simulink model "CustomLidarSLAM"  (R2024a)
settings: Solver=VariableStepAuto  StartTime=0.0  StopTime=30  RelTol=1e-3
model workspace (MAT data in the model file):
  IMUloc = [0 0 0]
values from neighbouring files (symbols this model uses):
  refPosesT = [timeVector, smoothRefPoses(:,3)]    [lidar_slam_project.m]    (also in lidar_slam_script.m)
  refPosesX = [timeVector, smoothRefPoses(:,1)]    [lidar_slam_project.m]    (also in lidar_slam_script.m)
  refPosesY = [timeVector, smoothRefPoses(:,2)]    [lidar_slam_project.m]    (also in lidar_slam_script.m)
undefined symbols (not defined in the file or in its folder): Sim3dSensor
libraries: vehdynlibsens x1, sim3dphyssensorlib x1, sim3dlib x1, sim3dautolib x1
settings Model: Creator=The MathWorks, Inc.  LastModifiedBy=FilippoOttaviani
settings SolverCC: AlgebraicLoopSolver=TrustRegion
settings DebuggingCC: UnconnectedInputMsg=warning  UnconnectedOutputMsg=warning  UnconnectedLineMsg=warning  SymbolicDimsDataTypeCodeGenerationDiagnostic=none
settings ModelReferenceCC: EnableRefExpFcnMdlSchedulingChecks=on
settings RTWCC: GPUComputeCapability=3.5  DLArmComputeVersion=19.05

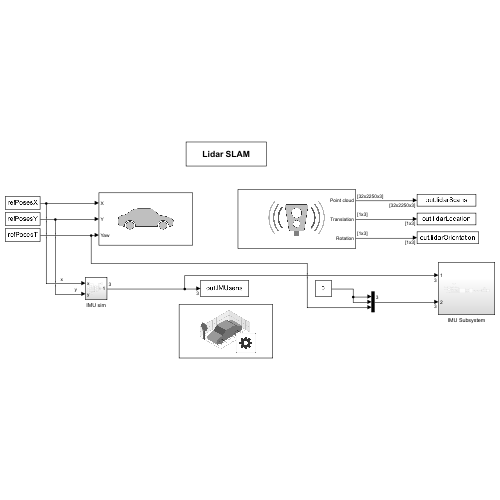
[thumbnail: Simulink's stored preview of the top-level diagram]
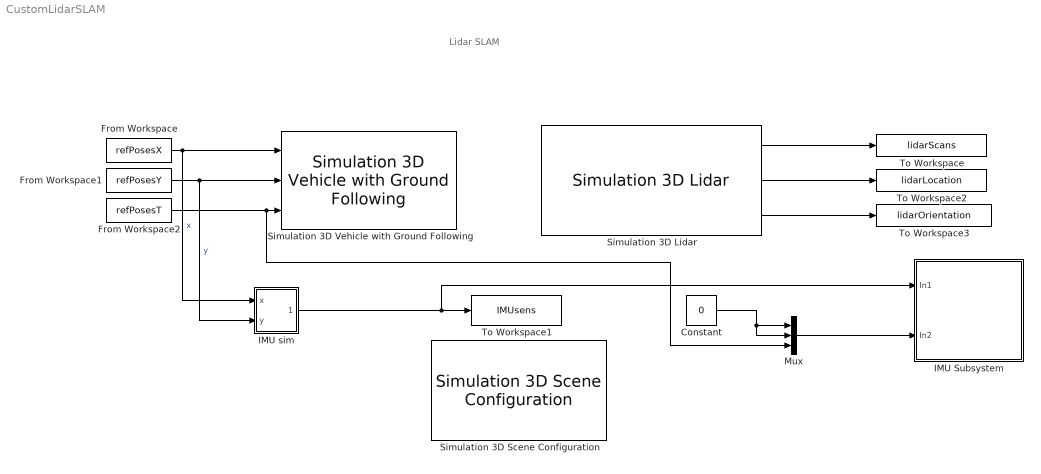
== system CustomLidarSLAM ==
  note: Lidar SLAM
  Constant : Constant  Value=0
  From Workspace : FromWorkspace  VariableName=refPosesX
  From Workspace1 : FromWorkspace  VariableName=refPosesY
  From Workspace2 : FromWorkspace  VariableName=refPosesT  Interpolate=off  OutputAfterFinalValue=Holding final value
  IMU Subsystem : Subsystem
  IMU sim : Subsystem
  Mux : Mux  Inputs=3
  Simulation 3D Lidar : sim3dphyssensorlib/Simulation 3D Lidar  Priority=1  sensorTag=Sim3dSensor�  sensorId=1  sensorName=Sim3dSensor�  vehTagList={'Scene Origin';'SimulinkVehicle1'}  vehTag=SimulinkVehicle1  mountLoc=Roof center  offsetFlag=off  tmountOffset=[0, 0, 0]  rmountOffset=[0, 0, 0]  DetectionRange=100  RangeResolution=0.02  VerticalFOV=40  VerticalResolution=1.25  HorizontalFOV=360  HorizontalResolution=0.16  DistanceOutportEnabled=off  ReflectivityOutportEnabled=off  SemanticOutportEnabled=off  TransformOutportEnabled=on  SampleTime=-1  mountPoint=[-0.25 0 1.57000005245209]  mountOrientation=[0 0 0]  aMode=5  ID=1
      settings: LibrarySourceBlock=sl3dlib/Simulation 3D/Sensors/Simulation 3D Lidar
  Simulation 3D Scene Configuration : sim3dlib/Simulation 3D Scene Configuration  Priority=0  ProjectFormat=Default Scenes  SceneDesc=US city block  ProjectName=C:\Program Files\MATLAB\R2024a\toolbox\shared\sim3d_projects\automotive_project_windows\UE\WindowsNoEditor\VehicleSimulation.exe  ScenePath=/Game/Maps/HwStrght  EnableOpenDRIVE=off  vehTagList={'Custom';'Scene Origin';'SimulinkVehicle1'}  vehTag=SimulinkVehicle1  FreeCameraInitialTranslation=[0, 0, 0]  FreeCameraDefaultInitialTranslation=[-6, 0, 2]  FreeCameraInitialRotation=[0, 0, 0]  FreeCameraDefaultInitialRotation=[0, -15, 0]  OpVisEn=off  Ts=1/60  EnableWindow=on  EnableRemoteAccess=off  EnableWeather=off  SunAzimuth=90  SunAltitude=40.0  EnableGeospatialSun=off  Latitude=0  Longitude=0  Date=2023-01-01  Time=10:30:00  GeoTimeZone=-5.0  SunDaylightSaving=off  wind=1  clouds=10  EnableVolumetricClouds=off  CloudCoverage=0  CloudAltitude=6  fog=0  rain=0  RaindropsEffect=off  SnowDensity=0  EnableGeospatial=off  UseTrueOrigin=off  OriginHeight=200  OriginLatitude=40.744652  OriginLongitude=-73.988864  MapStyle=Aerial  AdditionalAssetIDs=[]  UseAdvancedSunSky=off  SolarTime=11  TimeZone=-5  Day=21  Month=9  Year=2022  UseDaylightSavingTime=on  DSTStartDay=10  DSTStartMonth=3  DSTEndDay=3  DSTEndMonth=11  DSTSwitchHour=2  sensorTag=MainCamera2  sensorId=2  sensorName=MainCamera2  mountLoc=Origin  offsetFlag=off  tmountOffset=[0, 0, 0]  rmountOffset=[0, 0, 0]  HorizontalResolution=1280  VerticalResolution=720  HorizontalFOV=60  mountPoint=[0 0 0]  mountOrientation=[0 0 0]  aMode=3  ID=2  GeoTrigger=Inactive
      settings: LibrarySourceBlock=drivingsim3d/Simulation 3D Scene Configuration
  Simulation 3D Vehicle with Ground Following : sim3dautolib/Simulation 3D Vehicle with Ground Following  Priority=-1  PassVehMesh=Muscle car  MeshPath=/MathWorksSimulation/Vehicles/Muscle/Meshes/SK_MuscleCar.SK_MuscleCar  TrackWidth=1.9  WheelBase=3  WheelRadius=0.35  VehColor=Black  InitialPos=[refPosesX(1,2), refPosesY(1,2), 0]  InitialRot=[0, 0, refPosesT(1,2)]  ActorName=SimulinkVehicle1  SampleTime=-1  ActorType=SimulinkVehicle  ID=1  aMode=3  ActorTag=SimulinkVehicle1  CoordinateScheme=ISO  VehLightsControl=off  HeadlightColor=[ 1, 1, 1 ]  HighBeamIntensity=100000  LowBeamIntensity=60000  HighBeamConeAngle=70  LowBeamConeAngle=70  LeftHeadlightOrientation=[ 0, 0 ]  RightHeadlightOrientation=[ 0, 0 ]  BrakelightIntensity=500  ReverselightIntensity=500  SignallightIntensity=500  SignallightPeriod=1  SignalPulseWidth=50  TransformOutportEnabled=off
      settings: LibrarySourceBlock=drivingsim3d/Simulation 3D Vehicle with Ground Following
  To Workspace : ToWorkspace  VariableName=lidarScans  SaveFormat=Structure With Time  SampleTime=0.1
  To Workspace1 : ToWorkspace  VariableName=IMUsens  SaveFormat=Timeseries  SampleTime=-1
  To Workspace2 : ToWorkspace  VariableName=lidarLocation  SaveFormat=Structure With Time  SampleTime=0.1
  To Workspace3 : ToWorkspace  VariableName=lidarOrientation  SaveFormat=Structure With Time  SampleTime=0.1
  wires:
  From Workspace/1 -> IMU sim/1(x), Simulation 3D Vehicle with Ground Following/1  "x"
  From Workspace1/1 -> IMU sim/2(y), Simulation 3D Vehicle with Ground Following/2  "y"
  From Workspace2/1 -> Mux/3, Simulation 3D Vehicle with Ground Following/3
  Simulation 3D Lidar/2 -> To Workspace2/1
  Simulation 3D Lidar/3 -> To Workspace3/1
  Simulation 3D Lidar/1 -> To Workspace/1
  IMU sim/1(Out1) -> IMU Subsystem/1(In1), To Workspace1/1
  Mux/1 -> IMU Subsystem/2(In2)
  Constant/1 -> Mux/1, Mux/2

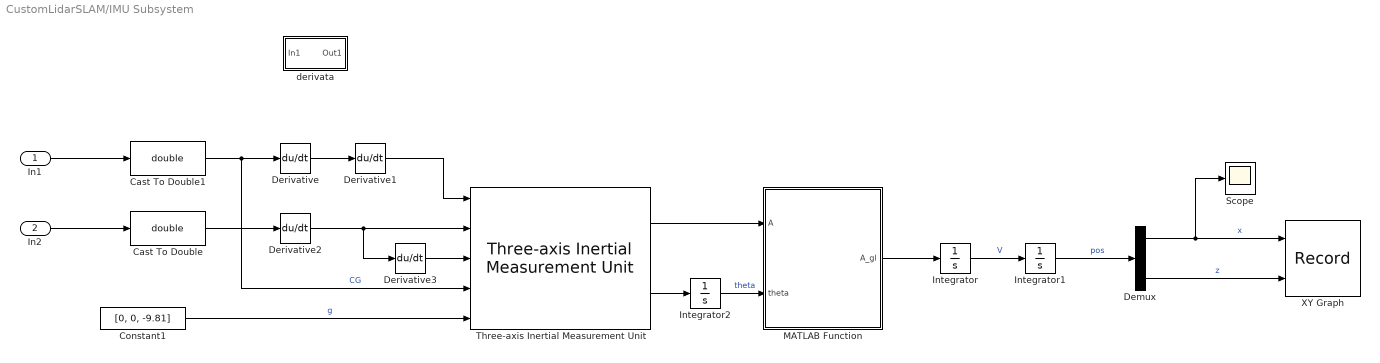
== system CustomLidarSLAM/IMU Subsystem ==
  In1 : Inport
  In2 : Inport  Port=2
  Cast To Double : DataTypeConversion  OutDataTypeStr=double  SaturateOnIntegerOverflow=off  RndMeth=Floor
  Cast To Double1 : DataTypeConversion  OutDataTypeStr=double  SaturateOnIntegerOverflow=off  RndMeth=Floor
  Constant1 : Constant  Value=[0, 0, -9.81]
  Demux : Demux  Outputs=3
  Derivative{,1..3} (4 alike) : Derivative
  Integrator : Integrator  InitialCondition=[0;0;0]
  Integrator1 : Integrator  InitialCondition=[0;0;0]
  Integrator2 : Integrator  InitialCondition=[0;0;0]
  MATLAB Function : MATLAB Function  TreatAsAtomicUnit=on
  Scope : Scope
  Three-axis Inertial Measurement Unit : vehdynlibsens/Three-axis Inertial Measurement Unit  units=Metric (MKS)  imu=[0;0;0]  i_Ts=0  dtype_a=off  w_a=190  z_a=0.707  a_sf_cc=[1 0 0; 0 1 0; 0 0 1]  a_bias=[0 0 0]  a_sat="[-inf  -inf  -inf  inf inf inf]"  dtype_g=off  w_g=190  z_g=0.707  g_sf_cc=[1 0 0; 0 1 0; 0 0 1]  g_bias=[0 0 0]  g_sens=[0 0 0]  g_sat="[-inf  -inf  -inf  inf inf inf]"  i_rand=off  i_seeds=[23093 23094 23095 23096 23097 23098]  i_pow=[0.001 0.001 0.001 0.0001 0.0001 0.0001]  aMode=2
  XY Graph : Record  FileSettingsInternal="{\"entries\":[{\"content\":{\"excelSettings\":{\"content\":{},\"type\":\"Streamout.ExcelSettings\"}},\"type\":\"Streamout.FileSettingStorage\",\"uuid\":\"\"}],\"packageUris\":[\"http:\\/\\/schema.mathworks.com\\/mf0\\/streamout_blocks\\/R2020a\"],\"version\":\"1.0\"}"  Layout=[1 1]  SignalsInternal="{\"entries\":[{\"content\":{\"signals\":[{\"content\":{\"blockPath\":[],\"dimensions\":[1,1],\"domain\":\"\",\"lineColor\":\"#edb120\",\"lineWidth\":2,\"plots\":[ 1 ],\"port\":1,\"sid\":[\"\"],\"signalID\":1,\"signalName\":\"x\"},\"type\":\"RecordBlkView.Signal\",\"uuid\":\"\"},{\"content\":{\"blockPath\":[],\"dimensions\":[1,1],\"domain\":\"\",\"lineColor\":\"#7e2f8e\",\"lineWidth\":2,\"plots\":[ 1 ],\"port\":2,\"sid\":[\"\"],\"signalID\":2,\"signalName\":\"z\"},\"type\":\"RecordBlkView.Signal\",\"uuid\":\"\"}]},\"type\":\"RecordBlkView.InputSignals\",\"uuid\":\"\"}],\"packageUris\":[\"http:\\/\\/schema.mathworks.com\\/mf0\\/streamout_blocks\\/R2020a\"],\"version\":\"1.0\"}"  VisualizationBindings="{\"xyplotplugin\":{\"info\":[{\"series\":[{\"bindingParametersList\":[{\"parameter\":\"X-Axis\",\"signalID\":1,\"signalName\":\"x\"},{\"parameter\":\"Y-Axis\",\"signalID\":2,\"signalName\":\"z\"}],\"seriesID\":0}],\"subplotID\":1}]}}"  CompatibilityTag=XY
  derivata : Subsystem
  wires:
  Three-axis Inertial Measurement Unit/2 -> Integrator2/1
  Integrator2/1 -> MATLAB Function/2(theta)  "theta"
  Integrator/1 -> Integrator1/1  "V"
  Cast To Double/1 -> Derivative2/1
  Three-axis Inertial Measurement Unit/1 -> MATLAB Function/1(A)
  In2/1 -> Cast To Double/1
  Constant1/1 -> Three-axis Inertial Measurement Unit/5  "g"
  Integrator1/1 -> Demux/1  "pos"
  MATLAB Function/1(A_gl) -> Integrator/1
  Derivative2/1 -> Derivative3/1, Three-axis Inertial Measurement Unit/2
  Cast To Double1/1 -> Derivative/1, Three-axis Inertial Measurement Unit/4  "CG"
  In1/1 -> Cast To Double1/1
  Derivative3/1 -> Three-axis Inertial Measurement Unit/3
  Demux/1 -> Scope/1, XY Graph/1  "x"
  Derivative1/1 -> Three-axis Inertial Measurement Unit/1
  Derivative/1 -> Derivative1/1
  Demux/3 -> XY Graph/2  "z"

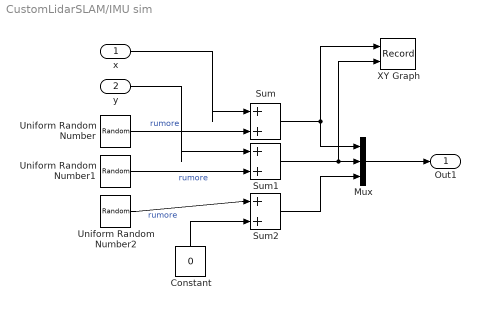
== system CustomLidarSLAM/IMU sim ==
  x : Inport
  y : Inport  Port=2
  Constant : Constant  Value=0
  Mux : Mux  Inputs=3
  Sum : Sum  Inputs=|++
  Sum1 : Sum  Inputs=|++
  Sum2 : Sum  Inputs=|++
  Uniform Random Number : UniformRandomNumber  Minimum=-0.1  Maximum=0.1  SampleTime=1
  Uniform Random Number1 : UniformRandomNumber  Minimum=-0.1  Maximum=0.1  SampleTime=1
  Uniform Random Number2 : UniformRandomNumber  Minimum=-0.1  Maximum=0.1  SampleTime=1
  XY Graph : Record  FileSettingsInternal="{\"entries\":[{\"content\":{\"excelSettings\":{\"content\":{},\"type\":\"Streamout.ExcelSettings\"}},\"type\":\"Streamout.FileSettingStorage\",\"uuid\":\"\"}],\"packageUris\":[\"http:\\/\\/schema.mathworks.com\\/mf0\\/streamout_blocks\\/R2020a\"],\"version\":\"1.0\"}"  Layout=[1 1]  SignalsInternal="{\"entries\":[{\"content\":{\"signals\":[{\"content\":{\"blockPath\":[],\"dimensions\":[1],\"domain\":\"\",\"lineColor\":\"#a2142f\",\"plots\":[ 1 ],\"port\":1,\"sid\":[\"\"],\"signalID\":1,\"signalName\":\"Sum\"},\"type\":\"RecordBlkView.Signal\",\"uuid\":\"\"},{\"content\":{\"blockPath\":[],\"dimensions\":[1],\"domain\":\"\",\"lineColor\":\"#139fff\",\"plots\":[ 1 ],\"port\":2,\"sid\":[\"\"],\"signalID\":2,\"signalName\":\"Sum1\"},\"type\":\"RecordBlkView.Signal\",\"uuid\":\"\"}]},\"type\":\"RecordBlkView.InputSignals\",\"uuid\":\"\"}],\"packageUris\":[\"http:\\/\\/schema.mathworks.com\\/mf0\\/streamout_blocks\\/R2020a\"],\"version\":\"1.0\"}"  VisualizationBindings="{\"xyplotplugin\":{\"info\":[{\"series\":[{\"bindingParametersList\":[{\"parameter\":\"X-Axis\",\"signalID\":1,\"signalName\":\"Sum\"},{\"parameter\":\"Y-Axis\",\"signalID\":2,\"signalName\":\"Sum1\"}],\"seriesID\":0}],\"subplotID\":1}]}}"  CompatibilityTag=XY
  Out1 : Outport
  wires:
  Constant/1 -> Sum2/2
  x/1 -> Sum/1
  Uniform Random Number1/1 -> Sum1/2  "rumore"
  Sum1/1 -> Mux/2, XY Graph/2
  Uniform Random Number2/1 -> Sum2/1  "rumore"
  Uniform Random Number/1 -> Sum/2  "rumore"
  Sum/1 -> XY Graph/1, Mux/1
  Sum2/1 -> Mux/3
  y/1 -> Sum1/1
  Mux/1 -> Out1/1

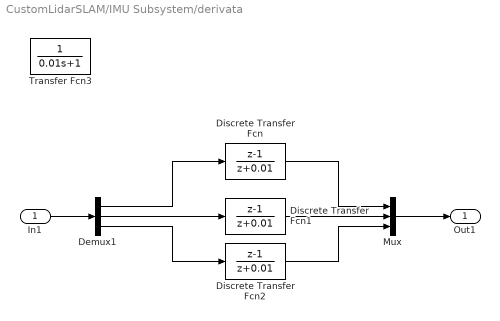
== system CustomLidarSLAM/IMU Subsystem/derivata ==
  In1 : Inport
  Demux1 : Demux  Outputs=3
  Discrete Transfer Fcn : DiscreteTransferFcn  Numerator=[1 -1]  Denominator=[1 0.01]
  Discrete Transfer Fcn1 : DiscreteTransferFcn  Numerator=[1 -1]  Denominator=[1 0.01]
  Discrete Transfer Fcn2 : DiscreteTransferFcn  Numerator=[1 -1]  Denominator=[1 0.01]
  Mux : Mux  Inputs=3
  Transfer Fcn3 : TransferFcn  Denominator=[0.01 1]
  Out1 : Outport
  wires:
  Demux1/1 -> Discrete Transfer Fcn/1
  Demux1/3 -> Discrete Transfer Fcn2/1
  Mux/1 -> Out1/1
  Demux1/2 -> Discrete Transfer Fcn1/1
  In1/1 -> Demux1/1
  Discrete Transfer Fcn/1 -> Mux/1
  Discrete Transfer Fcn1/1 -> Mux/2
  Discrete Transfer Fcn2/1 -> Mux/3

== matlab function CustomLidarSLAM/IMU Subsystem/MATLAB Function ==
  data: A input; A_gl output; theta input
function A_gl = conv2glob(A, theta)

    R_roll = [1 0 0;
        0 cos(theta(1)) -sin(theta(1))
        0 sin(theta(1)) cos(theta(1))];
    
    R_pitch = [cos(theta(2)) 0 sin(theta(2));
        0 1 0;
        -sin(theta(2)) 0 cos(theta(2))];
    
    R_yaw = [cos(theta(3)) -sin(theta(3)) 0
        sin(theta(3)) cos(theta(3)) 0
        0 0 1];

    R_tot = R_yaw*R_pitch*R_roll;
    %R_tot = R_roll * R_pitch * R_yaw

    A_gl = R_tot*A;
